simulink model "mech_clutch"  (Simulink 6.0)
settings: Solver=ode45  StartTime=0.0  StopTime=10.0  RelTol=1e-3  AbsTol=1e-6
PreLoadFcn:
  | load clutchparam.mat
values from neighbouring files (symbols this model uses):
  R = 5    [mech_fceng_init.m]
undefined symbols (not defined in the file or in its folder): be, bv, Ie, Iv, muk, mus
libraries: mblibv1 x12
settings Model: Creator=gwood  LastModifiedBy=batserve  ExtModeAutoUpdateStatusClock=off
settings DataIOCC: SignalLoggingName=logsOut
settings OptimizationCC: BooleanDataType=off
settings DebuggingCC: AlgebraicLoopMsg=none  CheckExecutionContextPreStartOutputMsg=on  CheckExecutionContextRuntimeOutputMsg=on  SolverPrmCheckMsg=none
settings HardwareCC: TargetUnknown=on

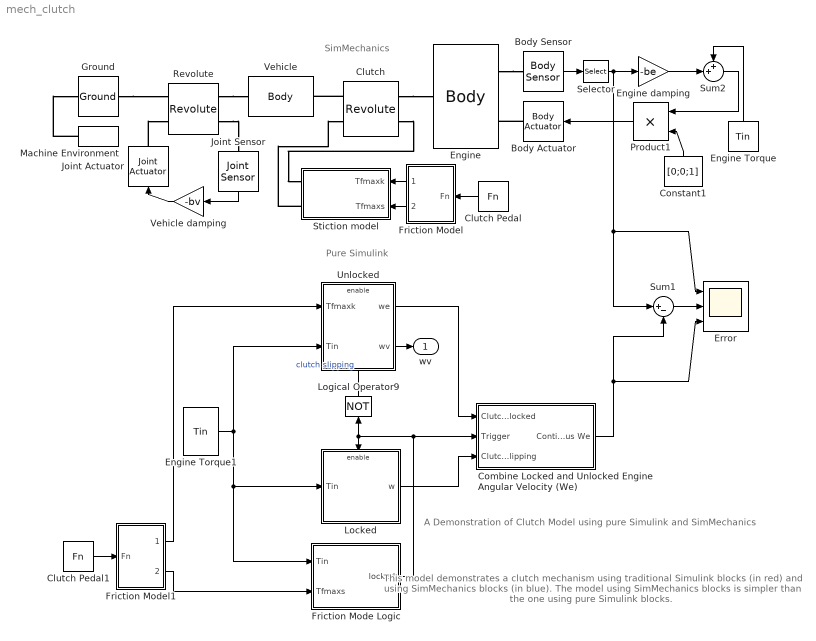
== system mech_clutch ==
  note: A Demonstration of Clutch Model using
      | pure Simulink and SimMechanics
  note: Pure Simulink
  note: SimMechanics
  note: This model demonstrates a clutch mechanism using traditional
      | Simulink blocks (in red) and using SimMechanics blocks (in blue).
      | The model using SimMechanics blocks is simpler than the one
      | using pure Simulink blocks.
  Body Actuator : mblibv1/Sensors &  Actuators/Body Actuator  Orientation=left  Opaque=on  PhysicalDomain=Mechanical  PortType=blob  ActuationStyle=Force  AngleUnits=deg  ArcVelocityUnits=deg/s  ArcAccelerationUnits=deg/s^2  CoordPositionUnits=m  VelocityUnits=m/s  AccelerationUnits=m/s^2  ForceUnits=N  TorqueUnits=N-m  ActiveIO=on  Width=3  DialogClass=MechanicalActuatorBlock  ReferenceFrame=Absolute (World)  Angle=off  CoordPosition=on  Force=off  Torque=on
  Body Sensor : mblibv1/Sensors &  Actuators/Body Sensor  Opaque=on  PhysicalDomain=Mechanical  PortType=blob  Muxed=on  Pose=off  Angle=on  AngleUnits=deg  ArcVelocity=on  ArcVelocityUnits=rad/s  ArcAcceleration=off  ArcAccelerationUnits=deg/s^2  CoordPosition=off  CoordPositionUnits=m  Velocity=off  VelocityUnits=m/s  Acceleration=off  AccelerationUnits=m/s^2  Quaternion=on  QuaternionDT=off  QuaternionDDT=off  QuaternionUnits=off  OutputVector=[ 3 ]  ActiveIO=on  Width=3  DialogClass=MechanicalSensorBlock  ReferenceFrame=Absolute (World)
  Clutch : mblibv1/Joints/Revolute  Orientation=left  PhysicalDomain=mechanical  SubClassName=Unknown  LeftPortType=blob  RightPortType=blob  LConnTagsString=__newl0|SA1  RConnTagsString=__newr0|SA1  NumSAPorts=2  CutJoint=off  MarkAsCut=off  Primitives=revolute  PrimitiveProps=R1$WORLD$[0 0 1]$revolute  DialogClass=JointBlock
  Clutch Pedal : FromWorkspace  Orientation=left  VariableName=Fn  SampleTime=0
  Clutch Pedal1 : FromWorkspace  VariableName=Fn  SampleTime=0
  Combine Locked and Unlocked Engine Angular Velocity (We) : Subsystem
  Constant1 : Constant  Orientation=up  Value=[0;0;1]
  Engine : mblibv1/Bodies/Body  PhysicalDomain=mechanical  SubClassName=Unknown  LeftPortType=workingframe  RightPortType=workingframe  LConnTagsString=CS1  RConnTagsString=CS2|CS3  DialogClass=MechanicalBodyBlock  Mass=1  MassUnits=kg  InertiaUnits=kg*m^2  Inertia=diag([0;0;Ie])  Shape=Cylinder  ShapeDims=[1 1]  ShapeUnits=m  ShapeUse=false  Density=1  DensityUnits=kg/m^3  DensityUse=false  CG=Left$CG$[0 0 0]$WORLD$WORLD$m$[0 0 0]$Euler X-Y-Z$deg$WORLD$false  WorkingFrames=Left$CS1$[0 0 0]$CG$CG$m$[0 0 0]$Euler X-Y-Z$deg$WORLD$true#Right$CS2$[0 0 0]$CG$CG$m$[0 0 0]$Euler X-Y-Z$deg$WORLD$true#Right$CS3$[0 0 0]$CG$CG$m$[0 0 0]$Euler X-Y-Z$deg$WORLD$true
  Engine Torque : FromWorkspace  Orientation=up  VariableName=Tin  SampleTime=0
  Engine Torque1 : FromWorkspace  VariableName=Tin  SampleTime=0
  Engine damping : Gain  Gain=-be  SaturateOnIntegerOverflow=on
  Error : Scope  NumInputPorts=3
      settings: TimeRange=10  YMin=0~-1e-014~0  YMax=0.8~5e-014~0.8
  Friction Model : Subsystem  Orientation=left
  Friction Model1 : Subsystem
  Friction Mode Logic : Subsystem
      mask Display: plot([-3 1 1 3 -1 -1],[-1 -1 1 1 1 -1],-4,-5,4,5)
  Ground : mblibv1/Bodies/Ground  Opaque=on  LeftPortType=env  RightPortType=workingframe  PhysicalDomain=Mechanical  DialogClass=GroundBlock  CoordPosition=[0 0 0]  CoordPositionUnits=m  StateVectorMgrId=-1  MachineId=[0 0]  ShowEnvPort=on
  Joint Actuator : mblibv1/Sensors &  Actuators/Joint Actuator  Orientation=up  Opaque=on  PhysicalDomain=Mechanical  PortType=blob  ActuationStyle=Force  AngleUnits=deg  ArcVelocityUnits=deg/s  ArcAccelerationUnits=deg/s^2  CoordPositionUnits=m  VelocityUnits=m/s  AccelerationUnits=m/s^2  ForceUnits=N  TorqueUnits=N-m  ActiveIO=on  Width=1  DialogClass=MechanicalActuatorBlock  Primitive=R1  ReferenceFrame=Absolute (INERTIAL)
  Joint Sensor : mblibv1/Sensors &  Actuators/Joint Sensor  Orientation=down  Opaque=on  PhysicalDomain=Mechanical  PortType=blob  Muxed=on  Pose=off  Angle=off  AngleUnits=deg  ArcVelocity=on  ArcVelocityUnits=rad/s  ArcAcceleration=off  ArcAccelerationUnits=deg/s^2  CoordPosition=on  CoordPositionUnits=m  Velocity=off  VelocityUnits=m/s  Acceleration=off  AccelerationUnits=m/s^2  Quaternion=on  QuaternionDT=off  QuaternionDDT=off  QuaternionUnits=off  OutputVector=[ 1 ]  ActiveIO=on  Width=1  DialogClass=MechanicalSensorBlock  Primitive=R1  Force=off  ForceUnits=N  Torque=off  TorqueUnits=N-m  ReferenceFrame=Absolute (INERTIAL)  ReactionSensedSide=Base  ReactionReferenceFrame=Absolute (World)  ReactionForce=off  ReactionForceUnits=N  ReactionMoment=off  ReactionMomentUnits=N-m
  Locked : Subsystem  TreatAsAtomicUnit=on
      mask Display: plot(-1,-6,6,12,[0 3],[3 3],[3 1 1 3], [1 1 5 5],[2 4 4 2],[4 4 2 2],[4 5],[3 3])
  Logical Operator9 : Logic  Orientation=up  Operator=NOT  Inputs=1
      mask Display: plot(0, -.25, 2., .5, [0 2 0 0], [-.5 0 .5 -.5],.2*cos(0:.1:2*pi)+2.2, .1*sin(0:.1:2*pi))
  Machine Environment : mblibv1/Bodies/Machine Environment  Tag=Factory ground  Orientation=left  DialogController=MECH.DialogSource  Opaque=on  PortType=env  PhysicalDomain=Mechanical  DialogTemplateClass=MECH.MachineEnvironment  SyncWhenCopied=off  Gravity=[0 0 0]  GravityUnits=m/s^2  GravityAsSignal=off  Dimensionality=3D Only  AnalysisType=Forward dynamics  LinearAssemblyTolerance=1e-3  LinearAssemblyToleranceUnits=m  AngularAssemblyTolerance=1e-3  AngularAssemblyToleranceUnits=rad  ConstraintSolverType=Stabilizing  ConstraintRelTolerance=1e-4  ConstraintAbsTolerance=1e-4  UseRobustSingularityHandling=off  StatePerturbationType=Fixed  PerturbationSize=1e-5  VisualizeMachine=on
  Product1 : Product  Orientation=left  SaturateOnIntegerOverflow=on  RndMeth=Zero  InputSameDT=on
  Revolute : mblibv1/Joints/Revolute  PhysicalDomain=mechanical  SubClassName=Unknown  LeftPortType=blob  RightPortType=blob  LConnTagsString=__newl0|SA1  RConnTagsString=__newr0|SA1  NumSAPorts=2  CutJoint=off  MarkAsCut=off  Primitives=revolute  PrimitiveProps=R1$WORLD$[0 0 1]$revolute  DialogClass=JointBlock
  Selector : Selector  Elements=3  InputPortWidth=3
  Stiction model : Subsystem  Orientation=left
  Sum1 : Sum  Inputs=|+-  SaturateOnIntegerOverflow=on  InputSameDT=on
  Sum2 : Sum  Inputs=++|  SaturateOnIntegerOverflow=on  InputSameDT=on
  Unlocked : Subsystem  TreatAsAtomicUnit=on
      mask Display: plot(-1,-2,6,8,[0 3],[3 3],[3 1 1 3], [1 1 5 5],[2 4 4 2],[4 4 2 2],[4 5],[3 3])
  Vehicle : mblibv1/Bodies/Body  PhysicalDomain=mechanical  SubClassName=Unknown  LeftPortType=workingframe  RightPortType=workingframe  LConnTagsString=CS1  RConnTagsString=CS2  DialogClass=MechanicalBodyBlock  Mass=0  MassUnits=kg  InertiaUnits=kg*m^2  Inertia=diag([0;0;Iv])  Shape=Cylinder  ShapeDims=[1 1]  ShapeUnits=m  ShapeUse=false  Density=1  DensityUnits=kg/m^3  DensityUse=false  CG=Left$CG$[0 0 0]$WORLD$WORLD$m$[0 0 0]$Euler X-Y-Z$deg$WORLD$false  WorkingFrames=Left$CS1$[0 0 0]$CG$CG$m$[0 0 0]$Euler X-Y-Z$deg$WORLD$true#Right$CS2$[0 0 0]$CG$CG$m$[0 0 0]$Euler X-Y-Z$deg$WORLD$true
  Vehicle damping : Gain  Orientation=left  Gain=-bv  SaturateOnIntegerOverflow=on
  wv : Outport  InitialOutput=0
  wires:
  Joint Sensor/1 -> Vehicle damping/1
  Vehicle damping/1 -> Joint Actuator/1
  Body Sensor/1 -> Selector/1
  Product1/1 -> Body Actuator/1
  Clutch Pedal/1 -> Friction Model/1(Fn)
  Friction Model/1(Tfmaxk) -> Stiction model/1(Tfmaxk)
  Friction Model/2(Tfmaxs) -> Stiction model/2(Tfmaxs)
  Selector/1 -> Engine damping/1, Error/1, Sum1/1
  Engine damping/1 -> Sum2/2
  Sum2/1 -> Product1/1
  Constant1/1 -> Product1/2
  Engine Torque1/1 -> Unlocked/2(Tin), Friction Mode Logic/1(Tin), Locked/1(Tin)
  Friction Model1/1(Tfmaxk) -> Unlocked/1(Tfmaxk)
  Unlocked/2(wv) -> wv/1
  Locked/1(w) -> Combine Locked and Unlocked Engine Angular Velocity (We)/3(Clutch slipping)
  Logical Operator9/1 -> Unlocked/Enable  "clutch slipping"
  Friction Model1/2(Tfmaxs) -> Friction Mode Logic/2(Tfmaxs)
  Clutch Pedal1/1 -> Friction Model1/1(Fn)
  Engine Torque/1 -> Sum2/1
  Unlocked/1(we) -> Combine Locked and Unlocked Engine Angular Velocity (We)/1(Clutch locked)
  Friction Mode Logic/1(locked) -> Combine Locked and Unlocked Engine Angular Velocity (We)/2(Trigger), Locked/Enable, Logical Operator9/1
  Combine Locked and Unlocked Engine Angular Velocity (We)/1(Continuous We) -> Error/3, Sum1/2
  Sum1/1 -> Error/2
  connections:
  Revolute/RConn1 -- Vehicle/LConn1
  Revolute/RConn2 -- Joint Sensor/LConn1
  Joint Actuator/RConn1 -- Revolute/LConn2
  Engine/RConn1 -- Body Sensor/LConn1
  Body Actuator/RConn1 -- Engine/RConn2
  Clutch/RConn1 -- Vehicle/RConn1
  Clutch/LConn1 -- Engine/LConn1
  Clutch/LConn2 -- Stiction model/RConn1
  Stiction model/RConn2 -- Clutch/RConn2
  Ground/RConn1 -- Revolute/LConn1
  Machine Environment/RConn1 -- Ground/LConn1

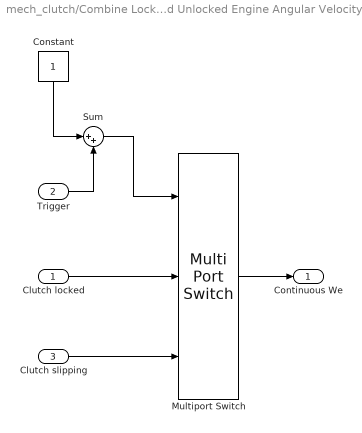
== system mech_clutch/Combine Locked and Unlocked Engine Angular Velocity (We) ==
  Clutch locked : Inport  Port=1  LatchInput=off
  Trigger : Inport  Port=2  LatchInput=off
  Clutch slipping : Inport  Port=3  LatchInput=off
  Constant : Constant  Orientation=down
  Multiport Switch : MultiPortSwitch  Inputs=2  SaturateOnIntegerOverflow=on  InputSameDT=on
  Sum : Sum  Inputs=|++  SaturateOnIntegerOverflow=on  InputSameDT=on
  Continuous We : Outport
  wires:
  Constant/1 -> Sum/1
  Trigger/1 -> Sum/2
  Multiport Switch/1 -> Continuous We/1
  Clutch locked/1 -> Multiport Switch/2
  Clutch slipping/1 -> Multiport Switch/3
  Sum/1 -> Multiport Switch/1

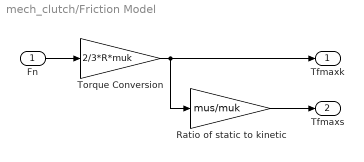
== system mech_clutch/Friction Model ==
  Fn : Inport  Port=1  LatchInput=off
  Ratio of static to kinetic : Gain  Gain=mus/muk  SaturateOnIntegerOverflow=on
  Torque Conversion : Gain  Gain=2/3*R*muk  SaturateOnIntegerOverflow=on
  Tfmaxk : Outport  InitialOutput=0
  Tfmaxs : Outport  Port=2  InitialOutput=0
  wires:
  Torque Conversion/1 -> Tfmaxk/1, Ratio of static to kinetic/1
  Fn/1 -> Torque Conversion/1
  Ratio of static to kinetic/1 -> Tfmaxs/1

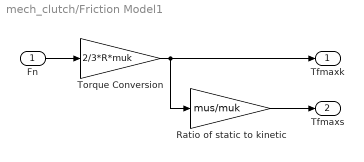
== system mech_clutch/Friction Model1 ==
  Fn : Inport  Port=1  LatchInput=off
  Ratio of static to kinetic : Gain  Gain=mus/muk  SaturateOnIntegerOverflow=on
  Torque Conversion : Gain  Gain=2/3*R*muk  SaturateOnIntegerOverflow=on
  Tfmaxk : Outport  InitialOutput=0
  Tfmaxs : Outport  Port=2  InitialOutput=0
  wires:
  Ratio of static to kinetic/1 -> Tfmaxs/1
  Fn/1 -> Torque Conversion/1
  Torque Conversion/1 -> Ratio of static to kinetic/1, Tfmaxk/1

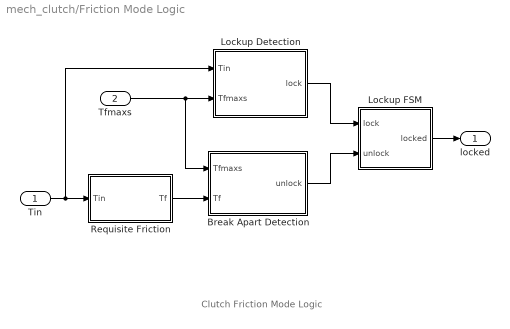
== system mech_clutch/Friction Mode Logic ==
  note: Clutch Friction Mode Logic
  Tin : Inport  Port=1  LatchInput=off
  Tfmaxs : Inport  Port=2  LatchInput=off
  Break Apart Detection : Subsystem
  Lockup Detection : Subsystem
  Lockup FSM : Subsystem
  Requisite Friction : Subsystem
  locked : Outport  InitialOutput=0
  wires:
  Lockup FSM/1(locked) -> locked/1
  Lockup Detection/1(lock) -> Lockup FSM/1(lock)
  Break Apart Detection/1(unlock) -> Lockup FSM/2(unlock)
  Requisite Friction/1(Tf) -> Break Apart Detection/2(Tf)
  Tfmaxs/1 -> Break Apart Detection/1(Tfmaxs), Lockup Detection/2(Tfmaxs)
  Tin/1 -> Requisite Friction/1(Tin), Lockup Detection/1(Tin)

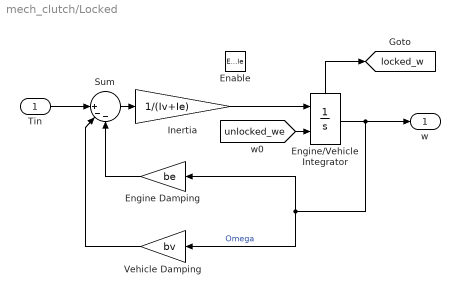
== system mech_clutch/Locked ==
  Tin : Inport  Port=1  LatchInput=off
  Enable : EnablePort  StatesWhenEnabling=reset
  Engine Damping : Gain  Orientation=left  Gain=be  SaturateOnIntegerOverflow=on
  Engine/Vehicle Integrator : Integrator  InitialConditionSource=external  ShowStatePort=on
  Inertia : Gain  Gain=1/(Iv+Ie)  SaturateOnIntegerOverflow=on
  Sum : Sum  Inputs=||+--  SaturateOnIntegerOverflow=on  InputSameDT=on
  Vehicle Damping : Gain  Orientation=left  Gain=bv  SaturateOnIntegerOverflow=on
  w : Outport  InitialOutput=0
  tag scope: locked_w=global
  wires:
  Vehicle Damping/1 -> Sum/2
  Inertia/1 -> Engine/Vehicle Integrator/1
  Engine Damping/1 -> Sum/3
  Engine/Vehicle Integrator/1 -> Vehicle Damping/1, Engine Damping/1, w/1  "Omega"
  Tin/1 -> Sum/1
  Sum/1 -> Inertia/1
  Engine/Vehicle Integrator/State -> [locked_w]
  [unlocked_we] -> Engine/Vehicle Integrator/2

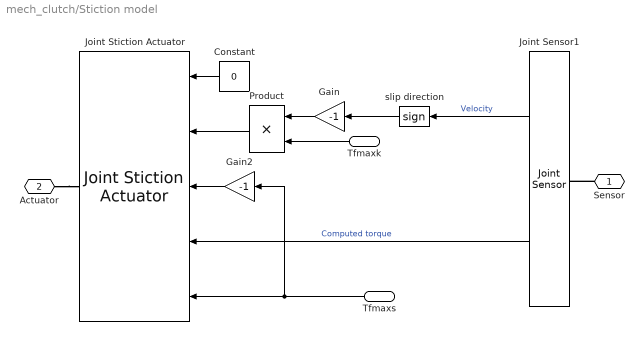
== system mech_clutch/Stiction model ==
  Tfmaxk : Inport  Orientation=left  Port=1  LatchInput=off
  Tfmaxs : Inport  Orientation=left  Port=2  LatchInput=off
  Constant : Constant  Orientation=left  Value=0
  Gain : Gain  Orientation=left  Gain=-1  SaturateOnIntegerOverflow=on
  Gain2 : Gain  Orientation=left  Gain=-1  SaturateOnIntegerOverflow=on
  Joint Sensor1 : mblibv1/Sensors &  Actuators/Joint Sensor  Orientation=left  Opaque=on  PhysicalDomain=Mechanical  PortType=blob  Muxed=off  Pose=off  Angle=off  AngleUnits=deg  ArcVelocity=on  ArcVelocityUnits=rad/s  ArcAcceleration=off  ArcAccelerationUnits=deg/s^2  CoordPosition=on  CoordPositionUnits=m  Velocity=off  VelocityUnits=m/s  Acceleration=off  AccelerationUnits=m/s^2  Quaternion=on  QuaternionDT=off  QuaternionDDT=off  QuaternionUnits=off  OutputVector=[ 1 1 ]  ActiveIO=on  Width=2  DialogClass=MechanicalSensorBlock  Primitive=R1  Force=off  ForceUnits=N  Torque=on  TorqueUnits=N-m  ReferenceFrame=Absolute (INERTIAL)  ReactionSensedSide=Base  ReactionReferenceFrame=Absolute (World)  ReactionForce=off  ReactionForceUnits=N  ReactionMoment=off  ReactionMomentUnits=N-m
  Joint Stiction Actuator : mblibv1/Sensors &  Actuators/Joint Stiction Actuator  Orientation=left  Opaque=on  PhysicalDomain=Mechanical  PortType=blob  ActuationStyle=Force  AngleUnits=deg  ArcVelocityUnits=deg/s  ArcAccelerationUnits=deg/s^2  CoordPositionUnits=m  VelocityUnits=m/s  AccelerationUnits=m/s^2  ForceUnits=N  TorqueUnits=N-m  ActiveIO=on  Width=5  DialogClass=EventActuatorBlock  Primitive=R1  FrictionalForceUnits=N-m  ExternalForceUnits=N-m  FrictionalTorqueUnits=N-m  ExternalTorqueUnits=N-m  LockingTolerance=1e-3
  Product : Product  Orientation=left  SaturateOnIntegerOverflow=on  RndMeth=Zero  InputSameDT=on
  slip direction : Signum  Orientation=left
  Sensor : PMIOPort  Orientation=left  Port=1  Side=Right
  Actuator : PMIOPort  Port=2  Side=Right
  wires:
  Joint Sensor1/1 -> slip direction/1  "Velocity"
  Product/1 -> Joint Stiction Actuator/2
  Gain/1 -> Product/1
  slip direction/1 -> Gain/1
  Gain2/1 -> Joint Stiction Actuator/3
  Tfmaxk/1 -> Product/2
  Joint Sensor1/2 -> Joint Stiction Actuator/4  "Computed torque"
  Constant/1 -> Joint Stiction Actuator/1
  Tfmaxs/1 -> Gain2/1, Joint Stiction Actuator/5
  connections:
  Sensor/RConn1 -- Joint Sensor1/LConn1
  Actuator/RConn1 -- Joint Stiction Actuator/RConn1

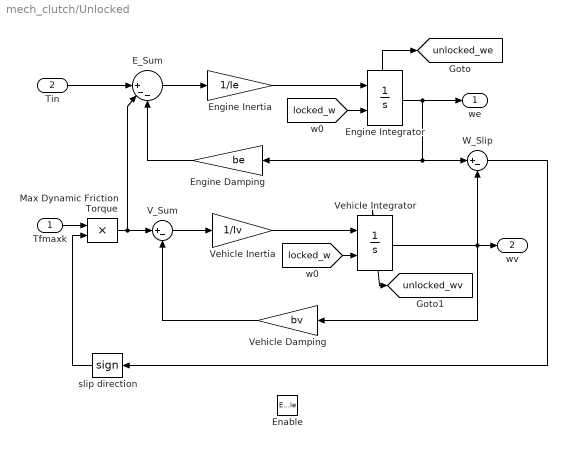
== system mech_clutch/Unlocked ==
  Tfmaxk : Inport  Port=1  LatchInput=off
  Tin : Inport  Port=2  LatchInput=off
  Enable : EnablePort  StatesWhenEnabling=reset
  E_Sum : Sum  Inputs=||+--  SaturateOnIntegerOverflow=on  InputSameDT=on
  Engine Damping : Gain  Orientation=left  Gain=be  SaturateOnIntegerOverflow=on
  Engine Inertia : Gain  Gain=1/Ie  SaturateOnIntegerOverflow=on
  Engine Integrator : Integrator  InitialConditionSource=external  ShowStatePort=on
  Max Dynamic Friction Torque : Product  SaturateOnIntegerOverflow=on  RndMeth=Zero  InputSameDT=on
  V_Sum : Sum  Inputs=|+-  SaturateOnIntegerOverflow=on  InputSameDT=on
  Vehicle Damping : Gain  Orientation=left  Gain=bv  SaturateOnIntegerOverflow=on
  Vehicle Inertia : Gain  Gain=1/Iv  SaturateOnIntegerOverflow=on
  Vehicle Integrator : Integrator  InitialConditionSource=external  ShowStatePort=on
  W_Slip : Sum  Inputs=|+-  SaturateOnIntegerOverflow=on  InputSameDT=on
  slip direction : Signum  Orientation=left
  we : Outport  InitialOutput=0
  wv : Outport  Port=2  InitialOutput=0
  tag scope: unlocked_we=global, unlocked_wv=global
  wires:
  Vehicle Integrator/1 -> W_Slip/2, wv/1, Vehicle Damping/1
  Vehicle Inertia/1 -> Vehicle Integrator/1
  [locked_w] -> Vehicle Integrator/2
  Vehicle Integrator/State -> [unlocked_wv]
  Tin/1 -> E_Sum/1
  [locked_w] -> Engine Integrator/2
  Engine Integrator/1 -> W_Slip/1, Engine Damping/1, we/1
  Engine Damping/1 -> E_Sum/3
  E_Sum/1 -> Engine Inertia/1
  Engine Inertia/1 -> Engine Integrator/1
  Engine Integrator/State -> [unlocked_we]
  W_Slip/1 -> slip direction/1
  slip direction/1 -> Max Dynamic Friction Torque/2
  Tfmaxk/1 -> Max Dynamic Friction Torque/1
  Max Dynamic Friction Torque/1 -> E_Sum/2, V_Sum/1
  Vehicle Damping/1 -> V_Sum/2
  V_Sum/1 -> Vehicle Inertia/1

== system mech_clutch/Friction Mode Logic/Break Apart Detection ==
  Tfmaxs : Inport  Port=1  LatchInput=off
  Tf : Inport  Port=2  LatchInput=off
  Abs : Abs  SaturateOnIntegerOverflow=on
  Relational Operator : RelationalOperator  InputSameDT=on
  unlock : Outport  InitialOutput=0
  wires:
  Tfmaxs/1 -> Relational Operator/2
  Abs/1 -> Relational Operator/1
  Relational Operator/1 -> unlock/1
  Tf/1 -> Abs/1

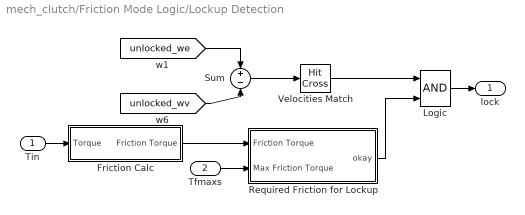
== system mech_clutch/Friction Mode Logic/Lockup Detection ==
  Tin : Inport  Port=1  LatchInput=off
  Tfmaxs : Inport  Port=2  LatchInput=off
  Friction Calc : Subsystem
  Logic : Logic
  Required Friction for Lockup : Subsystem
  Sum : Sum  Inputs=+-  SaturateOnIntegerOverflow=on  InputSameDT=on
  Velocities Match : HitCross
  lock : Outport  InitialOutput=0
  wires:
  Tin/1 -> Friction Calc/1(Torque)
  Sum/1 -> Velocities Match/1
  [unlocked_wv] -> Sum/2
  [unlocked_we] -> Sum/1
  Required Friction for Lockup/1(okay) -> Logic/2
  Logic/1 -> lock/1
  Velocities Match/1 -> Logic/1
  Tfmaxs/1 -> Required Friction for Lockup/2(Max Friction Torque)
  Friction Calc/1(Friction Torque) -> Required Friction for Lockup/1(Friction Torque)

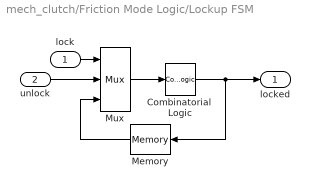
== system mech_clutch/Friction Mode Logic/Lockup FSM ==
  lock : Inport  Port=1  LatchInput=off
  unlock : Inport  Port=2  LatchInput=off
  Combinatorial  Logic : CombinatorialLogic  TruthTable=[0;1;0;0;1;1;1;0]
  Memory : Memory  Orientation=left
  Mux : Mux  Inputs=3
  locked : Outport  InitialOutput=0
  wires:
  Mux/1 -> Combinatorial  Logic/1
  lock/1 -> Mux/1
  unlock/1 -> Mux/2
  Combinatorial  Logic/1 -> Memory/1, locked/1
  Memory/1 -> Mux/3

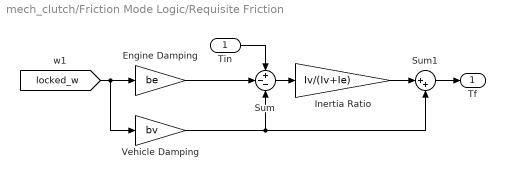
== system mech_clutch/Friction Mode Logic/Requisite Friction ==
  Tin : Inport  Port=1  LatchInput=off
  Engine Damping : Gain  Gain=be  SaturateOnIntegerOverflow=on
  Inertia Ratio : Gain  Gain=Iv/(Iv+Ie)  SaturateOnIntegerOverflow=on
  Sum : Sum  Inputs=+--  SaturateOnIntegerOverflow=on  InputSameDT=on
  Sum1 : Sum  Inputs=|++  SaturateOnIntegerOverflow=on  InputSameDT=on
  Vehicle Damping : Gain  Gain=bv  SaturateOnIntegerOverflow=on
  Tf : Outport  InitialOutput=0
  wires:
  Sum1/1 -> Tf/1
  Inertia Ratio/1 -> Sum1/1
  Tin/1 -> Sum/1
  Sum/1 -> Inertia Ratio/1
  Vehicle Damping/1 -> Sum1/2, Sum/3
  Engine Damping/1 -> Sum/2
  [locked_w] -> Engine Damping/1, Vehicle Damping/1

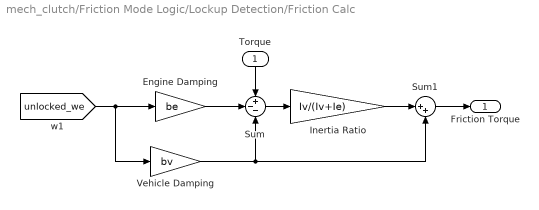
== system mech_clutch/Friction Mode Logic/Lockup Detection/Friction Calc ==
  Torque : Inport  Orientation=down  Port=1  LatchInput=off
  Engine Damping : Gain  Gain=be  SaturateOnIntegerOverflow=on
  Inertia Ratio : Gain  Gain=Iv/(Iv+Ie)  SaturateOnIntegerOverflow=on
  Sum : Sum  Inputs=+--  SaturateOnIntegerOverflow=on  InputSameDT=on
  Sum1 : Sum  Inputs=|++  SaturateOnIntegerOverflow=on  InputSameDT=on
  Vehicle Damping : Gain  Gain=bv  SaturateOnIntegerOverflow=on
  Friction Torque : Outport  InitialOutput=0
  wires:
  Sum1/1 -> Friction Torque/1
  Inertia Ratio/1 -> Sum1/1
  Torque/1 -> Sum/1
  Sum/1 -> Inertia Ratio/1
  Engine Damping/1 -> Sum/2
  Vehicle Damping/1 -> Sum/3, Sum1/2
  [unlocked_we] -> Vehicle Damping/1, Engine Damping/1

== system mech_clutch/Friction Mode Logic/Lockup Detection/Required Friction for Lockup ==
  Friction Torque : Inport  Port=1  LatchInput=off
  Max Friction Torque : Inport  Port=2  LatchInput=off
  Abs : Abs  SaturateOnIntegerOverflow=on
  Relational Operator : RelationalOperator  Operator=<=  InputSameDT=on
  okay : Outport  InitialOutput=0
  wires:
  Max Friction Torque/1 -> Relational Operator/2
  Abs/1 -> Relational Operator/1
  Relational Operator/1 -> okay/1
  Friction Torque/1 -> Abs/1
